simulink model "simulation"  (R2020b)
settings: Solver=VariableStepAuto  StartTime=0.0  StopTime=20  RelTol=1e-3
values from neighbouring files (symbols this model uses):
  Cm = [km*km*kr*kr/ra 0;0 0]    [script.m]
  get_C = matlabFunction(C)    [script.m]
  get_G = matlabFunction(G)    [script.m]
  get_inv_M = matlabFunction(inv_M)    [script.m]
  get_inv_M_hat = matlabFunction(inv_M_hat)    [script.m]
  get_M = matlabFunction(M)    [script.m]
  get_M_hat = matlabFunction(M_hat)    [script.m]
  theta0 = zeros(n_links, 1)    [script.m]
  theta_dot0 = zeros(n_links, 1)    [script.m]
  Vm = [kr*km/ra 0; 0 0]    [script.m]
settings Model: Creator=lucas  LastModifiedBy=lucas

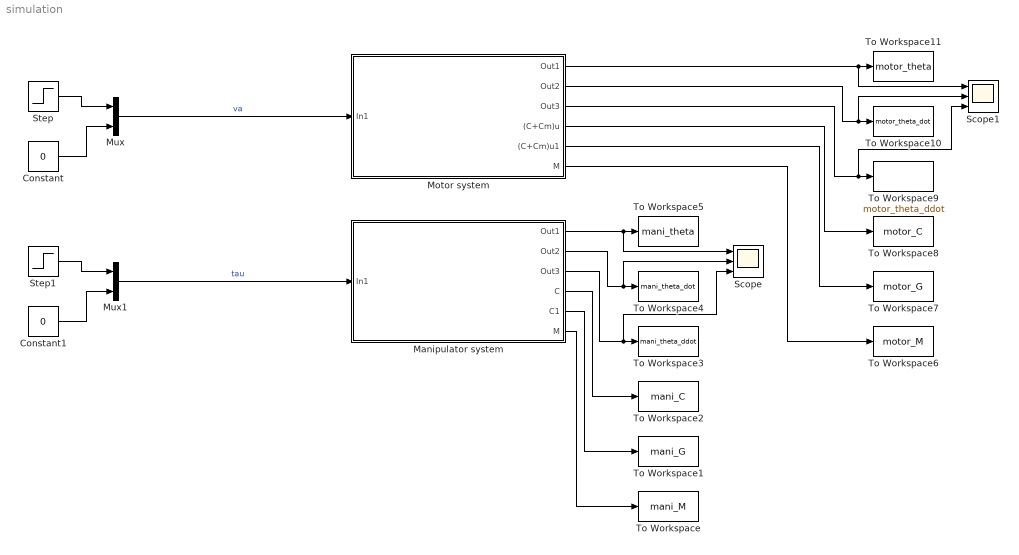
== system simulation ==
  Constant : Constant  Value=0
  Constant1 : Constant  Value=0
  Manipulator system : Subsystem
  Motor system : Subsystem
  Mux : Mux  Inputs=2
  Mux1 : Mux  Inputs=2
  Scope : Scope  NumInputPorts=3
  Scope1 : Scope  NumInputPorts=3
  Step : Step  After=0  SampleTime=0
  Step1 : Step  After=0  SampleTime=0
  To Workspace : ToWorkspace  VariableName=mani_M  SaveFormat=Timeseries  SampleTime=-1
  To Workspace1 : ToWorkspace  VariableName=mani_G  SaveFormat=Timeseries  SampleTime=-1
  To Workspace10 : ToWorkspace  VariableName=motor_theta_dot  SaveFormat=Timeseries  SampleTime=-1
  To Workspace11 : ToWorkspace  VariableName=motor_theta  SaveFormat=Timeseries  SampleTime=-1
  To Workspace2 : ToWorkspace  VariableName=mani_C  SaveFormat=Timeseries  SampleTime=-1
  To Workspace3 : ToWorkspace  VariableName=mani_theta_ddot  SaveFormat=Timeseries  SampleTime=-1
  To Workspace4 : ToWorkspace  VariableName=mani_theta_dot  SaveFormat=Timeseries  SampleTime=-1
  To Workspace5 : ToWorkspace  VariableName=mani_theta  SaveFormat=Timeseries  SampleTime=-1
  To Workspace6 : ToWorkspace  VariableName=motor_M  SaveFormat=Timeseries  SampleTime=-1
  To Workspace7 : ToWorkspace  VariableName=motor_G  SaveFormat=Timeseries  SampleTime=-1
  To Workspace8 : ToWorkspace  VariableName=motor_C  SaveFormat=Timeseries  SampleTime=-1
  To Workspace9 : ToWorkspace  VariableName=motor_theta_ddot  SaveFormat=Timeseries  SampleTime=-1
  wires:
  Step/1 -> Mux/1
  Constant/1 -> Mux/2
  Mux/1 -> Motor system/1(In1)  "va"
  Mux1/1 -> Manipulator system/1(In1)  "tau"
  Constant1/1 -> Mux1/2
  Step1/1 -> Mux1/1
  Manipulator system/6(M) -> To Workspace/1
  Manipulator system/5(C1) -> To Workspace1/1
  Manipulator system/4(C) -> To Workspace2/1
  Manipulator system/3(Out3) -> Scope/3, To Workspace3/1
  Manipulator system/2(Out2) -> Scope/2, To Workspace4/1
  Manipulator system/1(Out1) -> Scope/1, To Workspace5/1
  Motor system/2(Out2) -> Scope1/2, To Workspace10/1
  Motor system/1(Out1) -> Scope1/1, To Workspace11/1
  Motor system/3(Out3) -> Scope1/3, To Workspace9/1
  Motor system/4((C+Cm)u) -> To Workspace8/1
  Motor system/5((C+Cm)u1) -> To Workspace7/1
  Motor system/6(M) -> To Workspace6/1

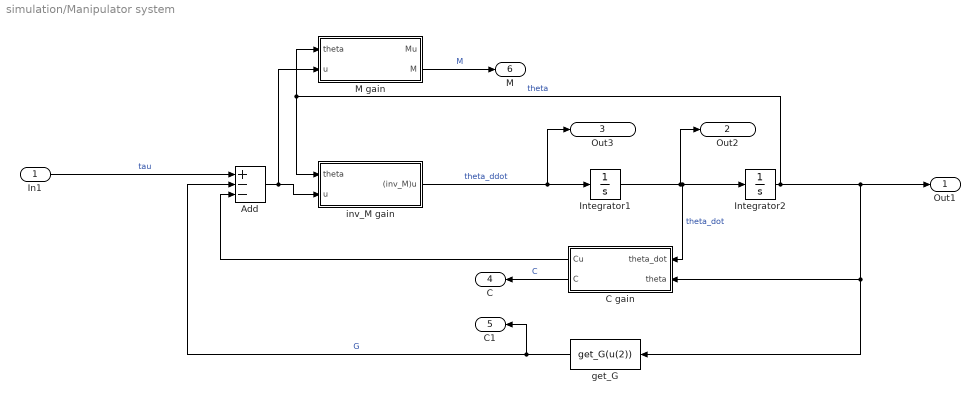
== system simulation/Manipulator system ==
  In1 : Inport
  Add : Sum  Inputs=+--
  C gain : Subsystem
  Integrator1 : Integrator  InitialCondition=theta_dot0
  Integrator2 : Integrator  InitialCondition=theta0
  M gain : Subsystem
  get_G : MATLABFcn  MATLABFcn=get_G(u(2))  Output1D=off
  inv_M gain : Subsystem
  Out1 : Outport
  Out2 : Outport  Port=2
  Out3 : Outport  Port=3
  C : Outport  Port=4
  C1 : Outport  Port=5
  M : Outport  Port=6
  wires:
  inv_M gain/1((inv_M)u) -> Integrator1/1, Out3/1  "theta_ddot"
  Integrator1/1 -> C gain/1(theta_dot), Integrator2/1, Out2/1  "theta_dot"
  In1/1 -> Add/1  "tau"
  Integrator2/1 -> inv_M gain/1(theta), M gain/1(theta), get_G/1, C gain/2(theta), Out1/1  "theta"
  C gain/1(Cu) -> Add/3
  get_G/1 -> C1/1, Add/2  "G"
  Add/1 -> M gain/2(u), inv_M gain/2(u)
  C gain/2(C) -> C/1  "C"
  M gain/2(M) -> M/1  "M"

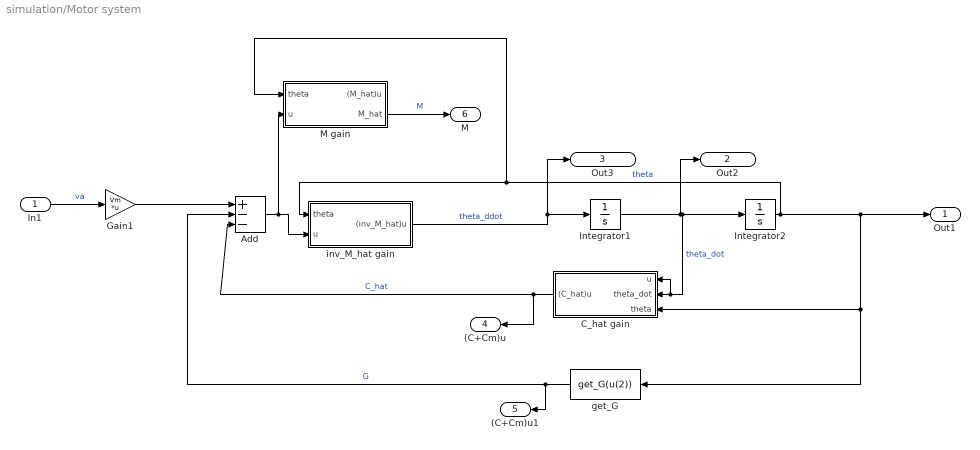
== system simulation/Motor system ==
  In1 : Inport
  Add : Sum  Inputs=+--
  C_hat gain : Subsystem
  Gain1 : Gain  Gain=Vm  Multiplication=Matrix(K*u) (u vector)
  Integrator1 : Integrator  InitialCondition=theta_dot0
  Integrator2 : Integrator  InitialCondition=theta0
  M gain : Subsystem
  get_G : MATLABFcn  MATLABFcn=get_G(u(2))  Output1D=off
  inv_M_hat gain : Subsystem
  Out1 : Outport
  Out2 : Outport  Port=2
  Out3 : Outport  Port=3
  (C+Cm)u : Outport  Port=4
  (C+Cm)u1 : Outport  Port=5
  M : Outport  Port=6
  wires:
  inv_M_hat gain/1((inv_M_hat)u) -> Integrator1/1, Out3/1  "theta_ddot"
  Integrator1/1 -> C_hat gain/2(theta_dot), C_hat gain/1(u), Integrator2/1, Out2/1  "theta_dot"
  In1/1 -> Gain1/1  "va"
  Gain1/1 -> Add/1
  Integrator2/1 -> inv_M_hat gain/1(theta), M gain/1(theta), get_G/1, C_hat gain/3(theta), Out1/1  "theta"
  C_hat gain/1((C_hat)u) -> (C+Cm)u/1, Add/3  "C_hat"
  get_G/1 -> (C+Cm)u1/1, Add/2  "G"
  Add/1 -> M gain/2(u), inv_M_hat gain/2(u)
  M gain/2(M_hat) -> M/1  "M"

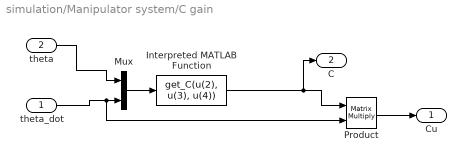
== system simulation/Manipulator system/C gain ==
  theta_dot : Inport
  theta : Inport  Port=2
  Interpreted MATLAB Function : MATLABFcn  MATLABFcn=get_C(u(2), u(3), u(4))  Output1D=off
  Mux : Mux  Inputs=2
  Product : Product  Multiplication=Matrix(*)
  Cu : Outport
  C : Outport  Port=2
  wires:
  Product/1 -> Cu/1
  Interpreted MATLAB Function/1 -> C/1, Product/1
  Mux/1 -> Interpreted MATLAB Function/1
  theta/1 -> Mux/1
  theta_dot/1 -> Product/2, Mux/2

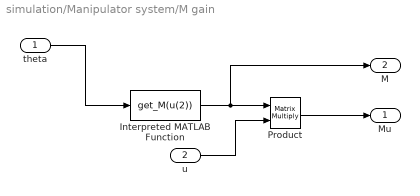
== system simulation/Manipulator system/M gain ==
  theta : Inport
  u : Inport  Port=2
  Interpreted MATLAB Function : MATLABFcn  MATLABFcn=get_M(u(2))  Output1D=off
  Product : Product  Multiplication=Matrix(*)
  Mu : Outport
  M : Outport  Port=2
  wires:
  Product/1 -> Mu/1
  Interpreted MATLAB Function/1 -> M/1, Product/1
  u/1 -> Product/2
  theta/1 -> Interpreted MATLAB Function/1

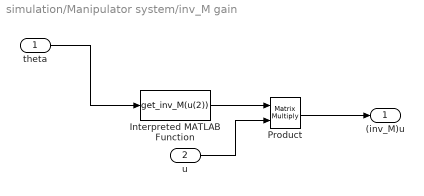
== system simulation/Manipulator system/inv_M gain ==
  theta : Inport
  u : Inport  Port=2
  Interpreted MATLAB Function : MATLABFcn  MATLABFcn=get_inv_M(u(2))  Output1D=off
  Product : Product  Multiplication=Matrix(*)
  (inv_M)u : Outport
  wires:
  Product/1 -> (inv_M)u/1
  Interpreted MATLAB Function/1 -> Product/1
  theta/1 -> Interpreted MATLAB Function/1
  u/1 -> Product/2

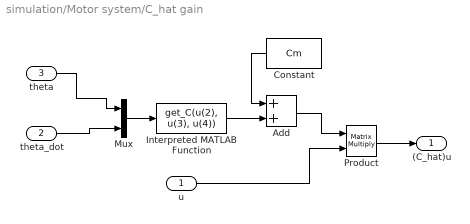
== system simulation/Motor system/C_hat gain ==
  u : Inport
  theta_dot : Inport  Port=2
  theta : Inport  Port=3
  Add : Sum
  Constant : Constant  Value=Cm
  Interpreted MATLAB Function : MATLABFcn  MATLABFcn=get_C(u(2), u(3), u(4))  Output1D=off
  Mux : Mux  Inputs=2
  Product : Product  Multiplication=Matrix(*)
  (C_hat)u : Outport
  wires:
  Product/1 -> (C_hat)u/1
  u/1 -> Product/2
  Interpreted MATLAB Function/1 -> Add/2
  Add/1 -> Product/1
  Constant/1 -> Add/1
  Mux/1 -> Interpreted MATLAB Function/1
  theta/1 -> Mux/1
  theta_dot/1 -> Mux/2

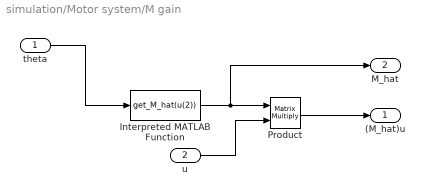
== system simulation/Motor system/M gain ==
  theta : Inport
  u : Inport  Port=2
  Interpreted MATLAB Function : MATLABFcn  MATLABFcn=get_M_hat(u(2))  Output1D=off
  Product : Product  Multiplication=Matrix(*)
  (M_hat)u : Outport
  M_hat : Outport  Port=2
  wires:
  Product/1 -> (M_hat)u/1
  Interpreted MATLAB Function/1 -> M_hat/1, Product/1
  u/1 -> Product/2
  theta/1 -> Interpreted MATLAB Function/1

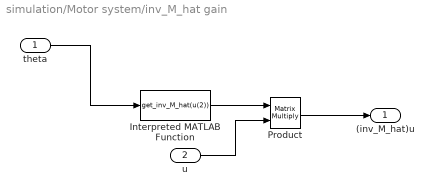
== system simulation/Motor system/inv_M_hat gain ==
  theta : Inport
  u : Inport  Port=2
  Interpreted MATLAB Function : MATLABFcn  MATLABFcn=get_inv_M_hat(u(2))  Output1D=off
  Product : Product  Multiplication=Matrix(*)
  (inv_M_hat)u : Outport
  wires:
  Product/1 -> (inv_M_hat)u/1
  Interpreted MATLAB Function/1 -> Product/1
  theta/1 -> Interpreted MATLAB Function/1
  u/1 -> Product/2
